simulink model "admire_bare_lin"  (Simulink 3.00)
settings: Solver=ode4  SolverMode=SingleTasking  StartTime=0.0  StopTime=500*0.02  FixedStep=0.02  RelTol=1e-3  AbsTol=1e-6
values from neighbouring files (symbols this model uses):
  x0 = [ max(eyp,zeros(n,1));max(-eyp,zeros(n,1));zeros(2*m,1)]    [LPwrap.m]
undefined symbols (not defined in the file or in its folder): dalpha_err, dalt_err, dbeta_err, dCl_beta, dCl_dai, dCl_day, dCl_dr, dCl_p, dCl_r, dCm_alpha, dCm_dei, dCm_dey, dCm_dne, dCm_q, dCn_beta, dCn_dna, dCn_dr, dCn_p, dCn_r, dCn_zero, dIxx, dIxz, dIyy, dIzz, dmass, dVt_err, dxcg, dycg, dzcg, u0new
libraries: simulink_extras x10
settings Model: SaveState=on  RTWOptions="-aLogVarNameModifier=\"rt_\" -aExtMode=0 -aRollThreshold=5 -aShowEliminatedStatements=1 -aRTWVerbose=1 -aInlineInvariantSignals=1 -aLocalBlockOutputs=1 -aInlineParameters=0"  RTWTemplateMakefile=grt_adm5p3.tmf  LastModifiedBy=lkh  ModifiedComment=nnt -- Mon Jun 05 13:08:11 2000 -- Version 3.42
settings Model: ModifiedHistory=|
  | nnt -- Mon Jun 05 13:08:11 2000 -- Version 3.42
  | 
  | 
  | nnt -- Mon Jun 05 11:01:33 2000 -- Version 3.41
  | 
  | 
  | nnt -- Mon Jun 05 10:57:40 2000 -- Version 3.40
  | 
  | 
  | nnt -- Mon Jun 05 10:56:46 2000 -- Version 3.39
  | 
  | 
  | hkg -- Thu Apr 13 16:38:30 2000 -- Version 3.38
  | Bug fix: all rate limiters were set with the canard parameters, now they get individual settings..
  | 
  | hkg -- Thu Apr 13 10:24:31 2000 -- Version 3.37
  | Inserted 3.0 version number in Level 1, changed month to April.
  | 
  | hkg -- Tue Apr 11 10:36:55 2000 -- Version 3.36
  | dtz re-connected
  | 
  | hkg -- Tue Apr 11 10:28:52 2000 -- Version 3.35
  | Changed the roll force saturation to +-80 N
  | 
  | hkg -- Tue Apr 11 09:23:02 2000 -- Version 3.34
  | All signal generators on Level 1 are now set to sine wave
  | 
  | hkg -- Mon Apr 10 15:03:16 2000 -- Version 3.33
  | New names for the RL_choice blocks
  | 
  | fosimadmin -- Mon Apr 10 13:44:14 2000 -- Version 3.32
  | Hkg actually. Nothing special
  | 
  | hkg -- Fri Apr 07 14:32:16 2000 -- Version 3.31
  | A few corrections to the names
  | 
  | hkg -- Fri Apr 07 14:16:55 2000 -- Version 3.30
  | Added unique names inside Saab and DASA rate limiters for left elevons, rudder and
  | leading-edge flaps.
  | hkg -- Fri Apr 07 14:04:35 2000 -- Version 3.29
  | Added unique names inside SAAB and DASA rate limiters for canard and right outer and
  | inner elevons.
  | hkg -- Thu Apr 06 17:23:24 2000 -- Version 3.28
  | Inserted unique names for rate limiters and multiport switches in the rate limiter selection blocks.
  | hkg -- Thu Apr 06 16:09:22 2000 -- Version 3.27
  | Disconnected dtz again. Chosen grt_adm5p3.tmf as template makefile. Code generation seems to work.
  | hyd -- Tue Mar 28 15:20:39 2000 -- Version 3.26
  | hyd -- Tue Mar 28 14:28:32 2000 -- Version 3.25
  | hyd -- Tue Mar 28 11:30:24 2000 -- Version 3.24
  | hyd -- Mon Mar 27 15:22:27 2000 -- Version 3.23
  | hyd -- Mon Mar 27 13:42:12 2000 -- Version 3.22
  | hyd -- Mon Mar 27 10:51:54 2000 -- Version 3.21
  | hyd -- Fri Mar 24 13:18:05 2000 -- Version 3.20
  | hyd -- Fri Mar 24 12:50:02 2000 -- Version 3.19
  | hyd -- Fri Mar 24 11:54:23 2000 -- Version 3.18
  | hyd -- Thu Mar 23 15:20:42 2000 -- Version 3.17
  | hyd -- Thu Mar 23 15:17:54 2000 -- Version 3.16
  | hyd -- Wed Mar 22 09:38:49 2000 -- Version 3.15
  | hyd -- Tue Mar 21 14:06:08 2000 -- Version 3.14
  | hyd -- Mon Mar 20 14:42:54 2000 -- Version 3.13
  | hyd -- Wed Mar 15 13:37:48 2000 -- Version 3.12
  | hyd -- Wed Mar 15 12:35:54 2000 -- Version 3.11
  | jnr -- Tue Mar 14 16:36:26 2000 -- Version 3.10
  | jnr -- Tue Mar 14 14:13:39 2000 -- Version 3.9
  | jnr -- Tue Mar 14 14:13:23 2000 -- Version 3.8
  | jnr -- Tue Mar 14 10:09:15 2000 -- Version 3.7
  | jnr -- Tue Mar 14 09:37:34 2000 -- Version 3.6
  | jnr -- Tue Mar 14 09:30:20 2000 -- Version 3.5
  | Add:
  | *proper stick gradients.
  | *correct gains for nz-control according to Åke Hydén.
  | *what transition region between q-control and nz-control is proper??
  | fll -- Fri Mar 03 09:53:48 2000 -- Version 3.4
  | changed name of "dtx" to "dty" (horizontal nozzle deflection)
  | fll -- Thu Mar 02 12:51:23 2000 -- Version 3.3
  | Reducesed the number of integrators to one in the longitudinal controller.
  | fll -- Thu Mar 02 12:30:52 2000 -- Version 3.2
  | Moved the blending function in the Nz and q controller.
  | fll -- Thu Mar 02 10:50:25 2000 -- Version 3.1
  | Changed input blocks to "Signal generator"
  | fll -- Thu Mar 02 10:50:25 2000 -- Version 3.0
  | Version 3.0 is modified according to comments from users

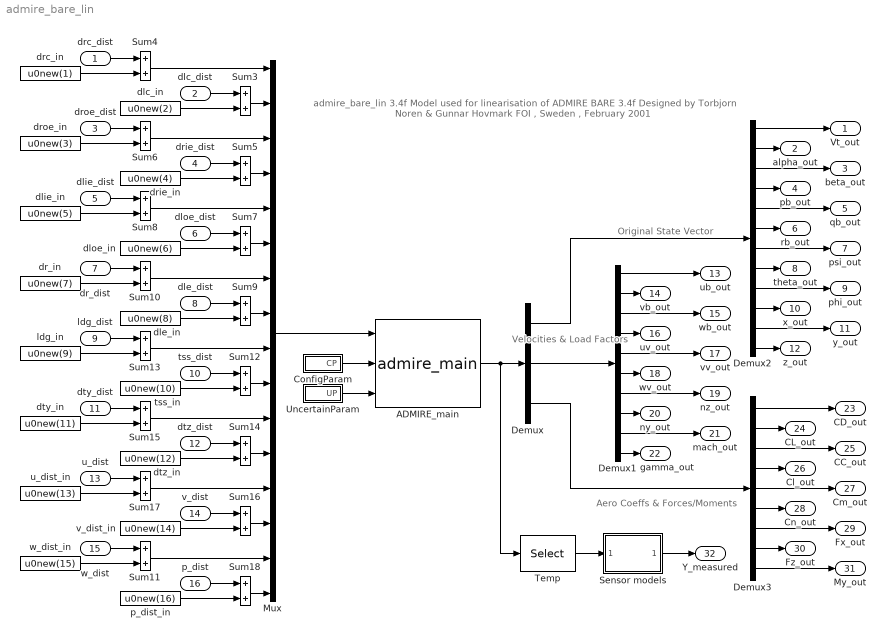
== system admire_bare_lin ==
  note: Original State Vector
  note: Velocities &
      | Load Factors
  note: Aero Coeffs &
      | Forces/Moments
  note: admire_bare_lin 3.4f
      | Model used for linearisation of ADMIRE BARE 3.4f
      | Designed by Torbjorn Noren & Gunnar Hovmark
      | FOI , Sweden , February 2001
  drc_dist : Inport  Port=1  PortWidth=-1  SampleTime=-1  DataType=auto
      settings: SignalType=auto
  dlc_dist : Inport  Port=2  PortWidth=-1  SampleTime=-1  DataType=auto
      settings: SignalType=auto
  droe_dist : Inport  Port=3  PortWidth=-1  SampleTime=-1  DataType=auto
      settings: SignalType=auto
  drie_dist : Inport  Port=4  PortWidth=-1  SampleTime=-1  DataType=auto
      settings: SignalType=auto
  dlie_dist : Inport  Port=5  PortWidth=-1  SampleTime=-1  DataType=auto
      settings: SignalType=auto
  dloe_dist : Inport  Port=6  PortWidth=-1  SampleTime=-1  DataType=auto
      settings: SignalType=auto
  dr_dist : Inport  Port=7  PortWidth=-1  SampleTime=-1  DataType=auto
      settings: SignalType=auto
  dle_dist : Inport  Port=8  PortWidth=-1  SampleTime=-1  DataType=auto
      settings: SignalType=auto
  ldg_dist : Inport  Port=9  PortWidth=-1  SampleTime=-1  DataType=auto
      settings: SignalType=auto
  tss_dist : Inport  Port=10  PortWidth=-1  SampleTime=-1  DataType=auto
      settings: SignalType=auto
  dty_dist : Inport  Port=11  PortWidth=-1  SampleTime=-1  DataType=auto
      settings: SignalType=auto
  dtz_dist : Inport  Port=12  PortWidth=-1  SampleTime=-1  DataType=auto
      settings: SignalType=auto
  u_dist : Inport  Port=13  PortWidth=-1  SampleTime=-1  DataType=auto
      settings: SignalType=auto
  v_dist : Inport  Port=14  PortWidth=-1  SampleTime=-1  DataType=auto
      settings: SignalType=auto
  w_dist : Inport  Port=15  PortWidth=-1  SampleTime=-1  DataType=auto
      settings: SignalType=auto
  p_dist : Inport  Port=16  PortWidth=-1  SampleTime=-1  DataType=auto
      settings: SignalType=auto
  ADMIRE_main : S-Function  FunctionName=admire_main  Parameters=x0bare dx0bare  PortCounts=[]  SFunctionModules=''
      mask Type: ADMIRE C-code block
      mask Description:
      | Main block describing the ADMIRE.
      | To use HELP, start any Internet browser.
      mask Help:
      | The aircraft it self is a C-code file that calculates the dynamics of the structure and the air surrounding it.<br>
      | The simulation requires an initial vector of values called x0 containing the following variables.<br><br>
      | 
      | Vt_init     --     initial airspeed.                        [m/s]<br>
      | alpha_init --    initial angle of attack.             [rad]<br>
      | beta_init    --   initial angle of sideslip.            [rad]<br>
      | pb_init     --     initial roll angular rate.             [rad/s]<br>
      | qb_init     --     initial pitch angular rate.          [rad/s]<br>
      | rb_init       --    initial yaw angular rate.           [rad/s]<br>
      | psi_init      --    initial euler angles (azimuth)    [rad]<br>
      | theta_init   --   initial (elevation)                      [rad]<br>
      | phi_init      --   initial (bank)                             [rad]<br>
      | xv_init      --    initial x position in Fv                [m]<br>
      | yv_init        --  initial y                                     [m]<br>
      | zv_init       --   initial z                                     [m]<br>
      mask Display:
      | plot([18 12 3 2 2 8 11],[7 4 1 1 2 8 11])
      | plot([13 11 13 15 15 13],[12 11 16 17 13 12])
      | plot([15 17 20 23 30 17],[13 14 24 25 20 14])
      | plot([30 38 40 38 30],[19 31 32 22 19])
      | plot([38.5 41 36 22 41 43 36],[23 21 16 10 8 10 16])
      | plot([15 19 25 24 15],[7 9 9 8 7])
      | plot([8 11 13 14 9 8],[8 11 12 10 7 8])
      | plot([21 23],[9 10])
      | plot([30 31],[20 20.5])
  ConfigParam : Subsystem
  Demux : Demux  Outputs=[12 10 9]
  Demux1 : Demux  Outputs=10
  Demux2 : Demux  Outputs=12
  Demux3 : Demux  Outputs=9
  Mux : Mux  Inputs=16
      settings: DisplayOption=none
  Sensor models : Subsystem
      mask Display: disp('Sensors')
  Sum{3..18} (16 alike) : Sum  Inputs=++  SaturateOnIntegerOverflow=on
  Temp : Selector  Elements=[1:28]  InputPortWidth=31
  UncertainParam : Subsystem
      mask Display: plot([0 10 5 0],[0 0 8.6603 0])
  dlc_in : Constant  Value=u0new(2)
  dle_in : Constant  Value=u0new(8)
  dlie_in : Constant  Value=u0new(5)
  dloe_in : Constant  Value=u0new(6)
  dr_in : Constant  Value=u0new(7)
  drc_in : Constant  Value=u0new(1)
  drie_in : Constant  Value=u0new(4)
  droe_in : Constant  Value=u0new(3)
  dty_in : Constant  Value=u0new(11)
  dtz_in : Constant  Value=u0new(12)
  ldg_in : Constant  Value=u0new(9)
  p_dist_in : Constant  Value=u0new(16)
  tss_in : Constant  Value=u0new(10)
  u_dist_in : Constant  Value=u0new(13)
  v_dist_in : Constant  Value=u0new(14)
  w_dist_in : Constant  Value=u0new(15)
  Vt_out : Outport  Port=1
  alpha_out : Outport  Port=2
  beta_out : Outport  Port=3
  pb_out : Outport  Port=4
  qb_out : Outport  Port=5
  rb_out : Outport  Port=6
  psi_out : Outport  Port=7
  theta_out : Outport  Port=8
  phi_out : Outport  Port=9
  x_out : Outport  Port=10
  y_out : Outport  Port=11
  z_out : Outport  Port=12
  ub_out : Outport  Port=13
  vb_out : Outport  Port=14
  wb_out : Outport  Port=15
  uv_out : Outport  Port=16
  vv_out : Outport  Port=17
  wv_out : Outport  Port=18
  nz_out : Outport  Port=19
  ny_out : Outport  Port=20
  mach_out : Outport  Port=21
  gamma_out : Outport  Port=22
  CD_out : Outport  Port=23
  CL_out : Outport  Port=24
  CC_out : Outport  Port=25
  Cl_out : Outport  Port=26
  Cm_out : Outport  Port=27
  Cn_out : Outport  Port=28
  Fx_out : Outport  Port=29
  Fz_out : Outport  Port=30
  My_out : Outport  Port=31
  Y_measured : Outport  Port=32
  wires:
  Sum3/1 -> Mux/2
  ConfigParam/1(CP) -> ADMIRE_main/2
  UncertainParam/1(UP) -> ADMIRE_main/3
  Mux/1 -> ADMIRE_main/1
  Demux/2 -> Demux1/1
  Demux/1 -> Demux2/1
  Demux/3 -> Demux3/1
  Demux2/2 -> alpha_out/1
  Demux2/4 -> pb_out/1
  Demux2/6 -> rb_out/1
  Demux2/8 -> theta_out/1
  Demux2/10 -> x_out/1
  Demux2/12 -> z_out/1
  Demux2/1 -> Vt_out/1
  Demux2/3 -> beta_out/1
  Demux2/5 -> qb_out/1
  Demux2/7 -> psi_out/1
  Demux2/9 -> phi_out/1
  Demux2/11 -> y_out/1
  Demux1/2 -> vb_out/1
  Demux1/4 -> uv_out/1
  Demux1/6 -> wv_out/1
  Demux1/8 -> ny_out/1
  Demux1/10 -> gamma_out/1
  Demux1/1 -> ub_out/1
  Demux1/3 -> wb_out/1
  Demux1/5 -> vv_out/1
  Demux1/7 -> nz_out/1
  Demux1/9 -> mach_out/1
  Demux3/2 -> CL_out/1
  Demux3/4 -> Cl_out/1
  Demux3/6 -> Cn_out/1
  Demux3/8 -> Fz_out/1
  Demux3/1 -> CD_out/1
  Demux3/3 -> CC_out/1
  Demux3/5 -> Cm_out/1
  Demux3/7 -> Fx_out/1
  Demux3/9 -> My_out/1
  Sensor models/1(admire_sensed_out) -> Y_measured/1
  Temp/1 -> Sensor models/1(admire_out)
  ADMIRE_main/1 -> Demux/1, Temp/1
  drc_dist/1 -> Sum4/1
  drc_in/1 -> Sum4/2
  Sum4/1 -> Mux/1
  dlc_dist/1 -> Sum3/1
  dlc_in/1 -> Sum3/2
  Sum5/1 -> Mux/4
  droe_dist/1 -> Sum6/1
  droe_in/1 -> Sum6/2
  Sum6/1 -> Mux/3
  drie_dist/1 -> Sum5/1
  drie_in/1 -> Sum5/2
  Sum7/1 -> Mux/6
  dlie_dist/1 -> Sum8/1
  dlie_in/1 -> Sum8/2
  Sum8/1 -> Mux/5
  dloe_dist/1 -> Sum7/1
  dloe_in/1 -> Sum7/2
  Sum9/1 -> Mux/8
  dr_dist/1 -> Sum10/1
  dr_in/1 -> Sum10/2
  Sum10/1 -> Mux/7
  dle_dist/1 -> Sum9/1
  dle_in/1 -> Sum9/2
  Sum12/1 -> Mux/10
  ldg_dist/1 -> Sum13/1
  ldg_in/1 -> Sum13/2
  Sum13/1 -> Mux/9
  tss_dist/1 -> Sum12/1
  tss_in/1 -> Sum12/2
  Sum14/1 -> Mux/12
  dty_dist/1 -> Sum15/1
  dty_in/1 -> Sum15/2
  Sum15/1 -> Mux/11
  dtz_dist/1 -> Sum14/1
  dtz_in/1 -> Sum14/2
  Sum16/1 -> Mux/14
  u_dist/1 -> Sum17/1
  u_dist_in/1 -> Sum17/2
  Sum17/1 -> Mux/13
  v_dist/1 -> Sum16/1
  v_dist_in/1 -> Sum16/2
  Sum18/1 -> Mux/16
  w_dist/1 -> Sum11/1
  w_dist_in/1 -> Sum11/2
  Sum11/1 -> Mux/15
  p_dist/1 -> Sum18/1
  p_dist_in/1 -> Sum18/2

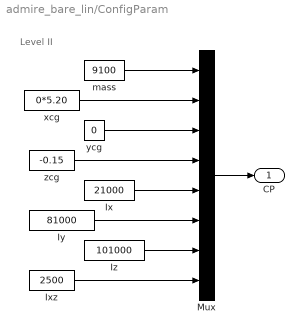
== system admire_bare_lin/ConfigParam ==
  note: Level II
  "Ix " : Constant  Value=21000
  "Ixz " : Constant  Value=2500
  "Iy " : Constant  Value=81000
  "Iz " : Constant  Value=101000
  Mux : Mux  Inputs=8
      settings: DisplayOption=none
  "mass " : Constant  Value=9100
  "xcg " : Constant  Value=0*5.20
  "ycg " : Constant  Value=0
  "zcg " : Constant  Value=-0.15
  CP : Outport  Port=1  InitialOutput=0
  wires:
  "mass "/1 -> Mux/1
  "xcg "/1 -> Mux/2
  "ycg "/1 -> Mux/3
  "zcg "/1 -> Mux/4
  "Ix "/1 -> Mux/5
  "Iy "/1 -> Mux/6
  "Iz "/1 -> Mux/7
  "Ixz "/1 -> Mux/8
  Mux/1 -> CP/1

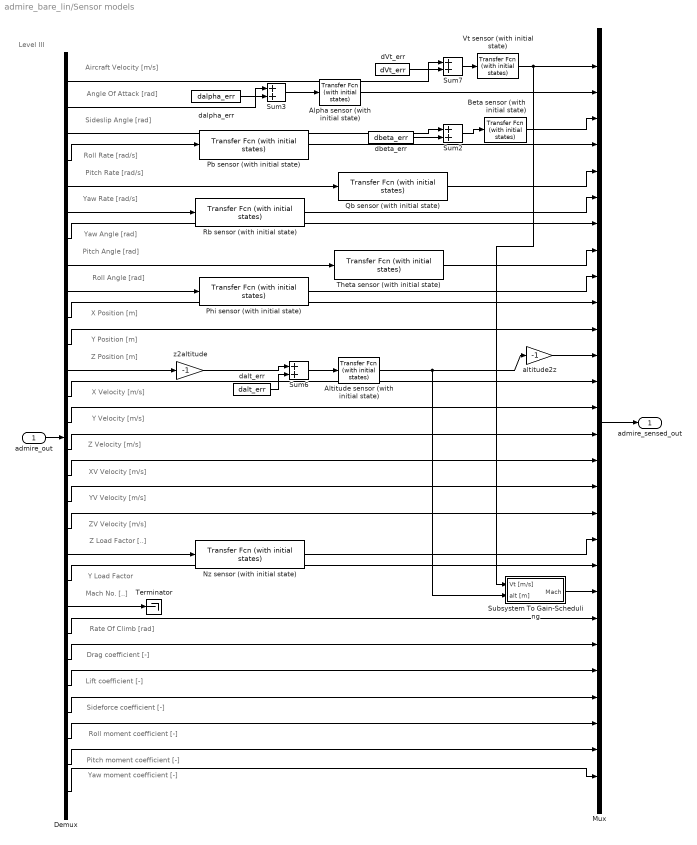
== system admire_bare_lin/Sensor models ==
  note: Aircraft Velocity [m/s]
  note: Angle Of Attack [rad]
  note: Sideslip Angle [rad]
  note: Roll Rate [rad/s]
  note: Pitch Rate [rad/s]
  note: Yaw Rate [rad/s]
  note: Yaw Angle [rad]
  note: Pitch Angle [rad]
  note: Roll Angle [rad]
  note: X Position [m]
  note: Y Position [m]
  note: Z Position [m]
  note: X Velocity [m/s]
  note: Y Velocity [m/s]
  note: Z Velocity [m/s]
  note: ZV Velocity [m/s]
  note: YV Velocity [m/s]
  note: XV Velocity [m/s]
  note: Z Load Factor [..]
  note: Y Load Factor
  note: Mach No. [..]
  note: Rate Of Climb [rad]
  note: Drag coefficient [-]
  note: Lift coefficient [-]
  note: Sideforce coefficient [-]
  note: Roll moment coefficient [-]
  note: Pitch moment coefficient [-]
  note: Yaw moment coefficient [-]
  note: Level III
  admire_out : Inport  Port=1  PortWidth=-1  SampleTime=-1  DataType=auto
      settings: SignalType=auto
  Alpha sensor (with initial state) : simulink_extras/Additional Linear/Transfer Fcn (with initial states)  N=[1]  D="[0.02  1]"  X0=x0(23)
  Altitude sensor (with initial state) : simulink_extras/Additional Linear/Transfer Fcn (with initial states)  N=[1]  D="[0.02  1]"  X0=x0(35)
  Beta sensor (with initial state) : simulink_extras/Additional Linear/Transfer Fcn (with initial states)  N=[1]  D="[0.02  1]"  X0=x0(24)
  Demux : Demux  Outputs=28
  Mux : Mux  Inputs=28
      settings: DisplayOption=none
  Nz sensor (with initial state) : simulink_extras/Additional Linear/Transfer Fcn (with initial states)  N=[0.0001903 0.005346 1]  D=[0.0004942 0.03082 1]  X0=[x0(36) x0(37)]
  Pb sensor (with initial state) : simulink_extras/Additional Linear/Transfer Fcn (with initial states)  N=[0.0001903 0.005346 1]  D=[0.0004942 0.03082 1]  X0=[x0(25) x0(26)]
  Phi sensor (with initial state) : simulink_extras/Additional Linear/Transfer Fcn (with initial states)  N=[1]  D=[0.00104 0.0323 1]  X0=[x0(33) x0(34)]
  Qb sensor (with initial state) : simulink_extras/Additional Linear/Transfer Fcn (with initial states)  N=[0.0001903 0.005346 1]  D=[0.0004942 0.03082 1]  X0=[x0(27) x0(28)]
  Rb sensor (with initial state) : simulink_extras/Additional Linear/Transfer Fcn (with initial states)  N=[0.0001903 0.005346 1]  D=[0.0004942 0.03082 1]  X0=[x0(29) x0(30)]
  Subsystem To Gain-Scheduling : Subsystem
  Sum{2..3,6..7} (4 alike) : Sum  Inputs=++  SaturateOnIntegerOverflow=on
  Terminator : Terminator
  Theta sensor (with initial state) : simulink_extras/Additional Linear/Transfer Fcn (with initial states)  N=[1]  D=[0.00104 0.0323 1]  X0=[x0(31) x0(32)]
  Vt sensor (with initial state) : simulink_extras/Additional Linear/Transfer Fcn (with initial states)  N=[1]  D="[0.02  1]"  X0=x0(22)
  altitude2z : Gain  Gain=-1  SaturateOnIntegerOverflow=off
  dVt_err : Constant  Value=dVt_err
  dalpha_err : Constant  Value=dalpha_err
  dalt_err : Constant  Value=dalt_err
  dbeta_err : Constant  Value=dbeta_err
  z2altitude : Gain  Gain=-1  SaturateOnIntegerOverflow=off
  admire_sensed_out : Outport  Port=1
  wires:
  Demux/24 -> Mux/24
  Demux/25 -> Mux/25
  Demux/26 -> Mux/26
  Demux/27 -> Mux/27
  Demux/28 -> Mux/28
  admire_out/1 -> Demux/1
  Qb sensor (with initial state)/1 -> Mux/5
  Demux/11 -> Mux/11
  Demux/13 -> Mux/13
  Demux/14 -> Mux/14
  Demux/5 -> Qb sensor (with initial state)/1
  Demux/4 -> Pb sensor (with initial state)/1
  Pb sensor (with initial state)/1 -> Mux/4
  Alpha sensor (with initial state)/1 -> Mux/2
  Demux/6 -> Rb sensor (with initial state)/1
  Rb sensor (with initial state)/1 -> Mux/6
  Demux/8 -> Theta sensor (with initial state)/1
  Theta sensor (with initial state)/1 -> Mux/8
  Demux/15 -> Mux/15
  Demux/16 -> Mux/16
  Demux/17 -> Mux/17
  Demux/18 -> Mux/18
  Demux/20 -> Mux/20
  Demux/22 -> Mux/22
  Demux/23 -> Mux/23
  Demux/21 -> Terminator/1
  dalpha_err/1 -> Sum3/2
  Demux/2 -> Sum3/1
  Sum3/1 -> Alpha sensor (with initial state)/1
  dbeta_err/1 -> Sum2/2
  Demux/3 -> Sum2/1
  Mux/1 -> admire_sensed_out/1
  Sum7/1 -> Vt sensor (with initial state)/1
  dVt_err/1 -> Sum7/2
  Demux/1 -> Sum7/1
  Vt sensor (with initial state)/1 -> Mux/1, Subsystem To Gain-Scheduling/1(Vt [m/s])
  Demux/9 -> Phi sensor (with initial state)/1
  Phi sensor (with initial state)/1 -> Mux/9
  Demux/7 -> Mux/7
  dalt_err/1 -> Sum6/2
  Sum6/1 -> Altitude sensor (with initial state)/1
  Demux/12 -> z2altitude/1
  z2altitude/1 -> Sum6/1
  Nz sensor (with initial state)/1 -> Mux/19
  Sum2/1 -> Beta sensor (with initial state)/1
  Beta sensor (with initial state)/1 -> Mux/3
  Demux/10 -> Mux/10
  Demux/19 -> Nz sensor (with initial state)/1
  altitude2z/1 -> Mux/12
  Altitude sensor (with initial state)/1 -> Subsystem To Gain-Scheduling/2(alt [m]), altitude2z/1
  Subsystem To Gain-Scheduling/1(Mach) -> Mux/21

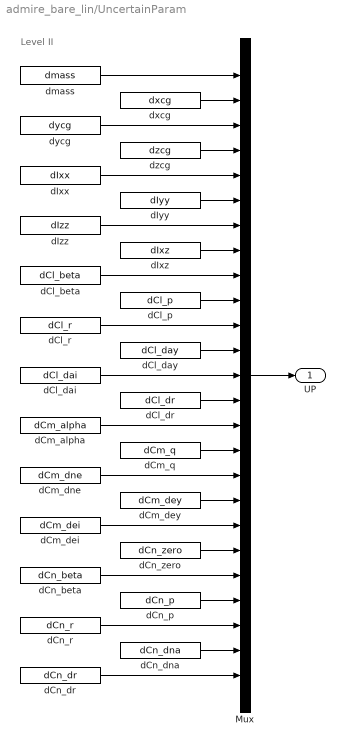
== system admire_bare_lin/UncertainParam ==
  note: Level II
  Mux : Mux  Inputs=25
      settings: DisplayOption=none
  "dCl_beta " : Constant  Value=dCl_beta
  "dCl_dai " : Constant  Value=dCl_dai
  dCl_day : Constant  Value=dCl_day
  "dCl_dr " : Constant  Value=dCl_dr
  "dCl_p " : Constant  Value=dCl_p
  "dCl_r " : Constant  Value=dCl_r
  "dCm_alpha " : Constant  Value=dCm_alpha
  "dCm_dei " : Constant  Value=dCm_dei
  "dCm_dey " : Constant  Value=dCm_dey
  "dCm_dne " : Constant  Value=dCm_dne
  "dCm_q " : Constant  Value=dCm_q
  "dCn_beta " : Constant  Value=dCn_beta
  dCn_dna : Constant  Value=dCn_dna
  "dCn_dr " : Constant  Value=dCn_dr
  "dCn_p " : Constant  Value=dCn_p
  "dCn_r " : Constant  Value=dCn_r
  dCn_zero : Constant  Value=dCn_zero
  dIxx : Constant  Value=dIxx
  dIxz : Constant  Value=dIxz
  "dIyy " : Constant  Value=dIyy
  "dIzz " : Constant  Value=dIzz
  "dmass " : Constant  Value=dmass
  dxcg : Constant  Value=dxcg
  "dycg " : Constant  Value=dycg
  "dzcg " : Constant  Value=dzcg
  UP : Outport  Port=1  InitialOutput=0
  wires:
  dCn_dna/1 -> Mux/24
  "dmass "/1 -> Mux/1
  "dycg "/1 -> Mux/3
  dxcg/1 -> Mux/2
  "dzcg "/1 -> Mux/4
  dIxx/1 -> Mux/5
  "dIyy "/1 -> Mux/6
  "dIzz "/1 -> Mux/7
  dIxz/1 -> Mux/8
  "dCl_beta "/1 -> Mux/9
  "dCl_p "/1 -> Mux/10
  "dCl_r "/1 -> Mux/11
  dCl_day/1 -> Mux/12
  "dCl_dai "/1 -> Mux/13
  "dCl_dr "/1 -> Mux/14
  "dCm_alpha "/1 -> Mux/15
  "dCm_q "/1 -> Mux/16
  "dCm_dey "/1 -> Mux/18
  dCn_zero/1 -> Mux/20
  "dCn_p "/1 -> Mux/22
  Mux/1 -> UP/1
  "dCm_dne "/1 -> Mux/17
  "dCm_dei "/1 -> Mux/19
  "dCn_beta "/1 -> Mux/21
  "dCn_dr "/1 -> Mux/25
  "dCn_r "/1 -> Mux/23

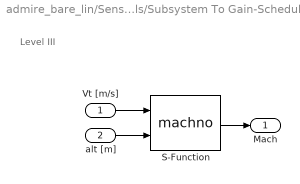
== system admire_bare_lin/Sensor models/Subsystem To Gain-Scheduling ==
  note: Level III
  Vt [m/s] : Inport  Port=1  PortWidth=-1  SampleTime=-1  DataType=auto
      settings: SignalType=auto
  alt [m] : Inport  Port=2  PortWidth=-1  SampleTime=-1  DataType=auto
      settings: SignalType=auto
  S-Function : S-Function  FunctionName=machno  PortCounts=[]  SFunctionModules=''
  Mach : Outport  Port=1
  wires:
  Vt [m/s]/1 -> S-Function/1
  S-Function/1 -> Mach/1
  alt [m]/1 -> S-Function/2
